simulink model "symulek"  (R2013a)
settings: Solver=ode45  StartTime=0.0  StopTime=10.0  RelTol=1e-3  AbsTol=1e-6
values from neighbouring files (symbols this model uses):
  a0 = Wn*2    (= 6)    [Skoki.m]    (also in symulek1.m = 1)
  a1 = Aw1*sqrt(2*g*h1max)/h1max    [Kaskady.m]    (also in Kaskady2.m; Skoki.m = 2*Wn*ksi(i); symulek1.m = 1; transmitacje.m)
  a2 = Aw2*sqrt(2*g*h2max)/h2max    [Kaskady.m]    (also in Kaskady2.m; Skoki.m = 1; transmitacje.m)
  b = 1    [Skoki.m]    (also in symulek1.m = 9)
  dirack = 1 - dirack    (= 0)    [Skoki.m]
  du = 1    [Skoki.m]    (also in symulek1.m)
  dx0 = 0    [Skoki.m]
  t0 = 1    [Kaskady.m]    (also in Kaskady2.m; Skoki.m = 0; symulek1.m; transmitacje.m)
  u0 = 0    [Skoki.m]    (also in symulek1.m)
  x0 = 0    [Skoki.m]    (also in symulek1.m)
settings Model: Creator=LAB320-1552  LastModifiedBy=LAB320-1552
settings DebuggingCC: SolverPrmCheckMsg=none

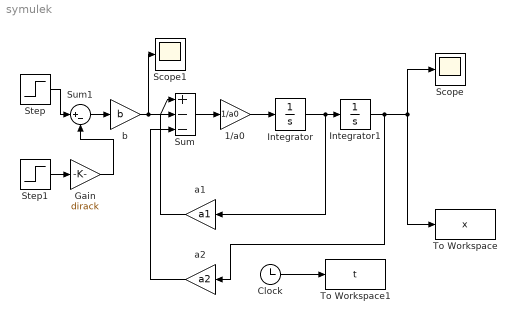
== system symulek ==
  1/a0 : Gain  Gain=1/a0
  Clock : Clock
  Gain : Gain  Gain=dirack
  Integrator : Integrator  InitialCondition=x0
  Integrator1 : Integrator  InitialCondition=dx0
  Scope : Scope
  Scope1 : Scope
  Step : Step  Time=t0  Before=u0  After=u0+du  SampleTime=0
  Step1 : Step  Time=t0+0.1  Before=u0  After=u0+du  SampleTime=0
  Sum : Sum  Inputs=|+--
  Sum1 : Sum  Inputs=|+-
  To Workspace : ToWorkspace  VariableName=x  SampleTime=-1
  To Workspace1 : ToWorkspace  VariableName=t  SampleTime=-1
  a1 : Gain  Gain=a1
  "a2 " : Gain  Gain=a2
  "b " : Gain  Gain=b
  wires:
  Step/1 -> Sum1/1
  Sum/1 -> 1/a0/1
  1/a0/1 -> Integrator/1
  Integrator/1 -> Integrator1/1, a1/1
  a1/1 -> Sum/2
  "b "/1 -> Scope1/1, Sum/1
  Clock/1 -> To Workspace1/1
  Integrator1/1 -> "a2 "/1, To Workspace/1, Scope/1
  "a2 "/1 -> Sum/3
  Sum1/1 -> "b "/1
  Step1/1 -> Gain/1
  Gain/1 -> Sum1/2
